simulink model "anti_windup_discrete"  (R2014b)
settings: Solver=ode45  StartTime=0.0  StopTime=20.0  RelTol=1e-3
values from neighbouring files (symbols this model uses):
  h = 0.14    [L9.m]    (also in anti_windup_analysis.m = 0.0918594343155; anti_windup_spring16.m = 0.1)
  Kp = 0.6*Ku    [PID_parameters_Carr_1986_example.m]    (also in anti_windup_analysis.m = 0.6667*Ku)
  N = 15    [anti_windup_analysis.m]    (also in anti_windup_spring16.m; tank_PID_tuning.m = 20)
  Td = Tu/8    (= 0.384999099705)    [PID_parameters_Carr_1986_example.m]    (also in anti_windup_analysis.m = 0.514358797205; anti_windup_spring16.m = 0.18125; tank_PID_tuning.m = 4.53125)
  Ti = Tu/2    (= 1.53999639882)    [PID_parameters_Carr_1986_example.m]    (also in anti_windup_analysis.m = 3.07999279764; anti_windup_spring16.m = 0.725; tank_PID_tuning.m = 18.125)
  Tt = 2*Ti    (= 6.15998559527)    [anti_windup_analysis.m]    (also in anti_windup_spring16.m = 0.3625)
  uHigh = 0.2    [anti_windup_analysis.m]    (also in anti_windup_spring16.m = 0.7)
  uLow = -0.2    [anti_windup_analysis.m]    (also in anti_windup_spring16.m = -0.7)
undefined symbols (not defined in the file or in its folder): i
settings Model: Creator=kjartan  LastModifiedBy=kjartan

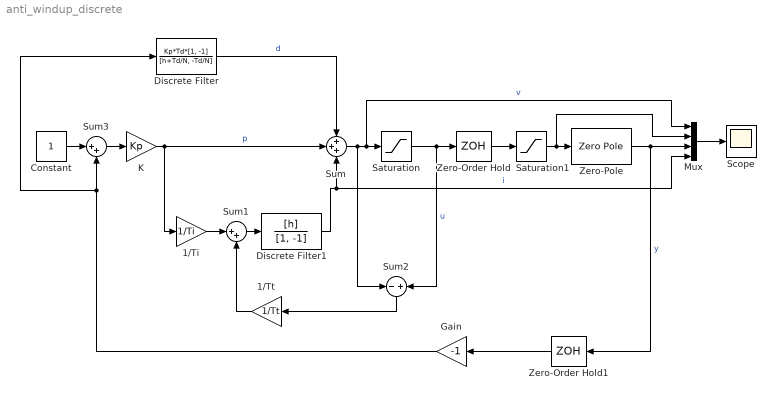
== system anti_windup_discrete ==
  1/Ti : Gain  Gain=1/Ti
  1/Tt : Gain  Gain=1/Tt
  Constant : Constant
  Discrete Filter : DiscreteFilter  Numerator=Kp*Td*[1, -1]  Denominator=[h+Td/N, -Td/N]  SampleTime=h
  Discrete Filter1 : DiscreteFilter  Numerator=[h]  Denominator=[1, -1]  SampleTime=h
  Gain : Gain  Gain=-1
  K : Gain  Gain=Kp
  Mux : Mux
  Saturation : Saturate  UpperLimit=uHigh  LowerLimit=uLow
  Saturation1 : Saturate  UpperLimit=uHigh  LowerLimit=uLow
  Scope : Scope
      settings: ShowLegends=on  TimeRange=20
  Sum : Sum  Inputs=+++
  Sum1 : Sum  Inputs=|++
  Sum2 : Sum  Inputs=-|+
  Sum3 : Sum  Inputs=|++
  Zero-Order Hold : ZeroOrderHold  SampleTime=h
  Zero-Order Hold1 : ZeroOrderHold  SampleTime=h
  Zero-Pole : ZeroPole  Zeros=[-3]  Poles=[0 -2 -1+2*i, -1-2*i]  Gain=[5]
  wires:
  Saturation/1 -> Zero-Order Hold/1, Sum2/2  "u"
  Sum/1 -> Mux/1, Saturation/1, Sum2/1  "v"
  Discrete Filter/1 -> Sum/1  "d"
  K/1 -> 1/Ti/1, Sum/2  "p"
  1/Ti/1 -> Sum1/1
  Sum1/1 -> Discrete Filter1/1
  Discrete Filter1/1 -> Sum/3, Mux/4  "i"
  Sum2/1 -> 1/Tt/1
  1/Tt/1 -> Sum1/2
  Zero-Pole/1 -> Zero-Order Hold1/1, Mux/3  "y"
  Constant/1 -> Sum3/1
  Sum3/1 -> K/1
  Mux/1 -> Scope/1
  Zero-Order Hold/1 -> Saturation1/1
  Saturation1/1 -> Mux/2, Zero-Pole/1
  Gain/1 -> Discrete Filter/1, Sum3/2
  Zero-Order Hold1/1 -> Gain/1
